simulink model "duty_cycle"  (R2021a)
settings: Solver=VariableStepAuto  StartTime=0.0  StopTime=0.01  RelTol=1e-3
libraries: spsPWMGeneratorDCDCLib x1, spsSawtoothGeneratorLib x1, spspowerguiLib x1
settings Model: Creator=Pichau  LastModifiedBy=Pichau

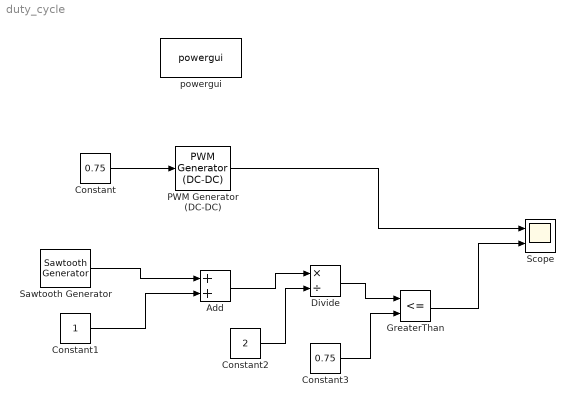
== system duty_cycle ==
  Add : Sum
  Constant : Constant  Value=0.75
  Constant1 : Constant
  Constant2 : Constant  Value=2
  Constant3 : Constant  Value=0.75
  Divide : Product  Inputs=*/
  GreaterThan : RelationalOperator  Operator=<=  OutDataTypeStr=boolean  RndMeth=Simplest
  PWM Generator (DC-DC) : spsPWMGeneratorDCDCLib/PWM Generator (DC-DC)  Fsw=5000  Ts=0
  Sawtooth Generator : spsSawtoothGeneratorLib/Sawtooth Generator  Freq=5e3  Phase=0  Ts=0
  Scope : Scope  NumInputPorts=2
  powergui : spspowerguiLib/powergui  Priority=1  SimulationMode=Continuous  SampleTime=50e-6  frequency=60  Iterations=50  frequencyindice=60  Pbase=100e6  ErrMax=1e-4  UnitsV=kV  UnitsW=MW  buscounter=0  FunctionMessages=off  echomessages=off  EnableUseOfTLC=off  CurrentSourceSwitches=off  DisableSnubberDevices=off  DisableRonSwitches=off  DisableVfSwitches=off  DisplayEquations=off  AutomaticDiscreteSolvers=off  SolverType=Tustin/Backward Euler (TBE)  Interpol=off  ExternalGateDelay=off  methode=off  Ts=100  x0status=blocks  SPID=on  SwTol=0  HookPort=off  NonlinearTolerance=1e-4  nMaxIteration=100  ContinueOnMaxIteration=off  RestoreLinks=warning  ResistiveCurrentMeasurement=off  Frange=[0:2:500]  Ylog=off  Xlog=on  ShowGrid=off  save=off  variable=ZData  structure=0  ZoomFFT=off  StartTime=0.0  cycles=1  DisplayStyle=1  fundamental=60  FreqAxis=off  MaxFrequency=1000  frequencyindicesteady=1  RmsSteady=1  display=off
  wires:
  Constant/1 -> PWM Generator (DC-DC)/1
  PWM Generator (DC-DC)/1 -> Scope/1
  Sawtooth Generator/1 -> Add/1
  Constant1/1 -> Add/2
  Add/1 -> Divide/1
  Constant2/1 -> Divide/2
  Divide/1 -> GreaterThan/1
  Constant3/1 -> GreaterThan/2
  GreaterThan/1 -> Scope/2
